simulink model "final_model_2"  (R2020a)
settings: Solver=VariableStepAuto  StartTime=0.0  StopTime=10.0  RelTol=1e-3
settings Model: Creator=hp  LastModifiedBy=hp

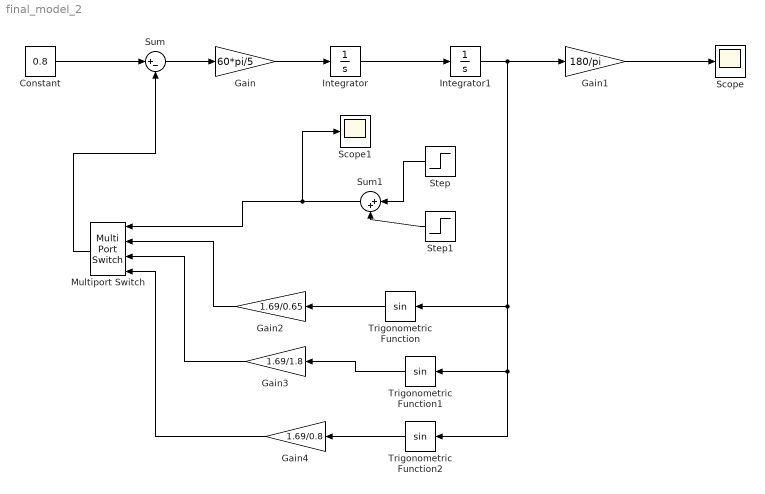
== system final_model_2 ==
  Constant : Constant  Value=0.8
  Gain : Gain  Gain=60*pi/5
  Gain1 : Gain  Gain=180/pi
  Gain2 : Gain  Gain=1.69/0.65
  Gain3 : Gain  Gain=1.69/1.8
  Gain4 : Gain  Gain=1.69/0.8
  Integrator : Integrator
  Integrator1 : Integrator
  Multiport Switch : MultiPortSwitch  DataPortOrder=Zero-based contiguous  zeroidx=on
  Scope : Scope
  Scope1 : Scope
  Step : Step  SampleTime=0
  Step1 : Step  Time=1.09  SampleTime=0
  Sum : Sum  Inputs=|+-
  Sum1 : Sum  Inputs=|++
  Trigonometric Function : Trigonometry
  Trigonometric Function1 : Trigonometry
  Trigonometric Function2 : Trigonometry
  wires:
  Constant/1 -> Sum/1
  Sum/1 -> Gain/1
  Gain/1 -> Integrator/1
  Integrator/1 -> Integrator1/1
  Multiport Switch/1 -> Sum/2
  Step/1 -> Sum1/1
  Step1/1 -> Sum1/2
  Sum1/1 -> Scope1/1, Multiport Switch/1
  Gain1/1 -> Scope/1
  Trigonometric Function/1 -> Gain2/1
  Gain2/1 -> Multiport Switch/2
  Integrator1/1 -> Trigonometric Function2/1, Trigonometric Function1/1, Trigonometric Function/1, Gain1/1
  Gain3/1 -> Multiport Switch/3
  Trigonometric Function1/1 -> Gain3/1
  Trigonometric Function2/1 -> Gain4/1
  Gain4/1 -> Multiport Switch/4
